simulink model "ModelCheck"  (R2023b)
(part 6 of 6)

0.023512 0.054235 0.056064 -0.038096 -0.013562 0.043326 -0.010964 -0.005109 -0.057211 -0.018286 0.060211 0.065341 0.047960 -0.020667 -0.013843 -0.001401 0.017310 0.045504 -0.018575 -0.019134 -0.073012 0.016395 0.009899 0.033708 0.094234 -0.024246 -0.000743 0.010348 -0.006107 0.049598 -0.022942 -0.003220 -0.049238 -0.012648 0.028773 0.020022 -0.039183 0.073379 0.031597 -0.023351 -0.013786 0.058244 0.016713 -0.017959 -0.057775 -0.004906 0.030304 0.004641 0.027545 -0.014616 0.021496 -0.041751 -0.039372 0.031919 0.045750 0.017093 -0.004608 0.025249 0.045686 -0.000110 -0.018566 -0.035737 0.054376 -0.085715 -0.000148 -0.019881 0.043376 -0.043883 -0.022043 0.072447 -0.013092 -0.047980 -0.047262 -0.008805 0.046933 0.023492 0.032296 -0.067832 -0.003275 0.008644 -0.024545 0.004619 -0.012919 -0.001176 0.038797 -0.014456 -0.088259 -0.035865 0.045722 -0.018662 0.008622 -0.099365 -0.003551 -0.026567 -0.030622 0.050041 -0.005362 0.011961 0.033541 0.036222 0.008774 -0.009115 0.031861 -0.021490 0.049896 0.031574 -0.039833 -0.009175;];

b_fc3=[-0.050248;0.019419;-0.007584;-0.004701;
    0.066879;0.008068;0.012271;0.037518;
    0.018469;0.025402;-0.030088;0.020672;
    -0.014795;-0.020354;0.026809;0.010165;
    -0.028667;0.012238;-0.033566;-0.018052;
    -0.023610;-0.019974;0.022028;0.011272;
    0.001126;-0.016021;-0.015038;-0.038405;
    0.003107;0.015127;0.001553;0.014676;
    0.026649;-0.002020;-0.015832;0.019317;
    0.008205;-0.062022;-0.022966;0.007499;
    -0.012638;0.018665;0.032723;0.014381;
    -0.037361;-0.013134;0.016202;0.023778;
    0.003392;0.012089;-0.057931;-0.030821;
    0.019307;-0.024789;-0.024829;-0.019109;
    -0.036828;0.024116;0.032070;-0.005278;
    -0.054152;0.020843;0.005430;-0.009851;
    -0.016264;0.019022;0.024571;-0.011725;
    0.033968;0.018459;-0.017238;0.003314;
    0.016000;-0.015041;-0.048086;-0.016735;
    0.009188;-0.026200;0.014782;-0.010735;
    -0.018216;-0.007501;-0.006561;-0.009650;
    -0.028159;-0.035850;-0.010736;-0.007596;
    0.006820;-0.022196;-0.052921;-0.029646;
    -0.015627;0.014437;-0.017289;-0.028943;
    -0.011719;0.020001;0.013502;-0.024150;
    0.009400;-0.006621;-0.006457;-0.015976;
    0.021786;-0.006809;0.011536;-0.012874;
    0.015784;-0.000610;-0.011105;0.015037;
    0.013845;-0.013274;0.018924;0.035682;
    -0.010498;0.017744;0.004284;0.020030;
    0.000363;-0.003400;0.006331;0.075977;
    -0.018280;-0.015513;0.109497;-0.013426;];

W_fc4=[0.026027 0.110741 0.161431 0.167392 -0.190671 -0.125685 0.075150 -0.155269 -0.087090 -0.055340 0.076587 -0.081340 0.184739 -0.070082 -0.028536 0.040011 -0.022169 0.022260 0.000044 -0.040060 0.028046 -0.006128 -0.162195 -0.045412 -0.012831 -0.101741 -0.034443 0.127086 -0.141235 0.051987 0.029246 0.041341 -0.091715 0.108888 -0.010136 -0.003129 -0.156203 0.134836 0.038879 0.151228 -0.068602 -0.142881 0.003074 0.030582 -0.045517 -0.032294 -0.069688 -0.081765 0.131343 0.110648 -0.016502 0.189732 -0.152022 0.043125 -0.052186 -0.011396 0.136952 0.048061 0.087187 0.001019 0.185365 0.001288 0.103990 -0.105580 -0.087727 -0.096446 -0.073437 -0.083990 -0.106592 -0.094862 0.073546 -0.133156 -0.002561 -0.065258 0.075292 0.155931 -0.231823 -0.016414 0.073010 0.082288 0.150805 0.052044 0.079674 -0.067201 -0.009314 -0.018984 0.198832 -0.178292 -0.113881 0.191550 0.192360 0.129858 0.168286 0.020856 0.161164 0.155435 -0.054277 -0.076461 0.091337 0.020808 0.179029 -0.004578 0.192330 -0.015879 -0.082812 0.225540 -0.163496 -0.075460 -0.052403 0.108064 -0.122821 -0.102711 -0.169872 -0.076572 -0.034603 -0.103318 -0.125369 -0.077881 0.127496 -0.017238 0.109801 0.112558 -0.065103 -0.194935 0.242926 -0.097697 0.013485 0.177124;0.159687 0.126462 -0.086977 0.048017 0.115216 -0.046373 -0.190716 -0.010674 -0.124673 -0.131871 0.094752 -0.085853 -0.038550 0.249178 0.018542 -0.173446 0.073181 -0.184545 0.103904 -0.047020 0.147135 0.233303 -0.018168 0.170688 -0.128298 0.044245 0.115063 -0.180727 0.096201 -0.242247 -0.019905 -0.078126 -0.085383 0.003224 0.222446 -0.110632 -0.070378 -0.035165 0.002250 -0.155158 0.110721 -0.178589 -0.146177 0.014449 -0.107264 0.105571 -0.092844 0.097968 0.004097 -0.247947 0.205642 0.016957 -0.175277 0.217190 0.088294 0.160585 0.178121 -0.081880 0.082925 -0.122988 0.027655 0.082715 -0.080247 0.094665 0.084331 -0.168889 -0.144491 0.055702 0.044761 -0.164660 0.160570 0.176872 -0.117555 0.053752 0.115425 0.153265 0.093910 0.052035 0.008975 -0.091821 -0.158360 -0.174010 0.097309 0.127758 0.144934 0.073049 0.194521 0.027616 0.040887 0.105044 -0.122287 0.107725 0.014322 -0.203017 0.010793 -0.133184 0.098581 -0.100807 -0.107960 0.033678 -0.071194 0.113878 0.096965 0.100678 -0.178719 0.126049 -0.164581 0.149564 -0.043040 -0.149966 0.154813 -0.144642 0.189624 0.032040 -0.085721 0.136431 0.131641 0.113282 0.026591 -0.148824 0.113943 0.055452 -0.002636 -0.007852 0.149575 0.161948 -0.066083 -0.198966;-0.092739 -0.169485 0.126114 -0.180247 -0.094097 -0.022461 0.000901 -0.089657 -0.095458 -0.215169 0.102442 -0.168352 0.135316 -0.057663 -0.135851 0.086314 0.133720 -0.056147 0.021493 0.205406 0.037576 0.047440 -0.102276 0.216004 0.147343 0.169350 0.195265 0.128172 -0.123537 0.056020 0.042814 -0.217024 -0.159612 -0.142414 0.079931 -0.212307 0.130910 0.066442 0.074539 -0.128386 -0.023330 -0.011075 0.044190 -0.151654 0.074232 0.159139 -0.233880 -0.057523 -0.157185 0.123466 -0.120281 -0.016502 -0.139356 0.026709 0.064551 0.113031 0.062139 -0.190568 -0.019484 0.088167 0.043900 -0.201632 -0.034114 0.045618 0.210745 -0.040332 -0.100856 0.164020 -0.023038 -0.168417 0.065491 -0.046767 -0.116580 0.177485 -0.128807 -0.037005 -0.157136 0.155910 -0.118527 0.134019 0.095050 -0.141623 -0.010149 0.157671 0.068934 0.211115 0.121864 0.204309 -0.080933 -0.023835 0.193535 -0.137080 0.060757 -0.029869 -0.085182 0.145462 0.159472 -0.191918 -0.239322 0.014231 -0.079560 0.109832 -0.014623 0.183315 -0.151255 -0.108035 -0.056916 0.180924 0.026579 0.064874 0.089399 -0.186550 0.163683 0.209722 -0.048261 -0.124964 0.139386 -0.144076 -0.131380 -0.190648 -0.059812 0.033392 -0.032087 -0.008788 -0.069460 0.186372 -0.149921 -0.186034;];

b_fc4=[-0.035603;-0.017302;-0.022000;];

output = zeros(3,1);

output(1) = x(1) + t*x_ddot;

output(2) = x(2) + t*y_ddot;

psi_dot = x(3) + t*psi_ddot;

output(3) = x(4) + t*psi_dot;

out1=tanh(W_fc1*U+b_fc1);

out2=tanh(W_fc2*out1+b_fc2);

out3=tanh(W_fc3*out2+b_fc3);

out4=W_fc4*out3+b_fc4;

% Output = out4;

% X_new = [Output(1,:); Output(2,:);Output(3,:); x(4:end,:)];

x_new = [output(1); output(2); psi_dot; output(3)];

end
